simulink model "ctrl_student_HIL.previous"  (R2015a)
settings: Solver=ode4  StartTime=0.0  StopTime=inf  FixedStep=0.01  RelTol=1e-3
(part 3 of 3)

== matlab function ctrl_student_HIL.previous/Transfer function ==
  data: s input; eta input; nu input; mu input; rx input; ry input; kp1 input; kp2 input; kp3 input; s_dot output; tau output; eta_d output; case_number input
function [s_dot, tau, eta_d] = maneuver(s, eta, nu, mu, rx, ry, kp1, kp2, kp3, case_number)
%% Constants
P_d = [2 0; 10 4];
K_p = diag([kp1+0.2 kp2+0.2 kp3+0.1]);
K_2 = 10*eye(3); K_2(3, 3) = K_2(3, 3) / 2;
U_max = 0.6548;

%% Parameters
% Rigid body and added mass
m = 14.79; 
I_z = 1.76; 
x_g = 0.0375; 
% y_g = 0.0;

X_u_dot = -2; 
Y_v_dot = -10; 
Y_r_dot = -0; 
N_r_dot = -1; 

% Max Values in Surge X, Sway Y and Yaw N
X_max = 1.03; %[N]
Y_max = 2.50; %[N]
N_max = 0.98; %[Nm]


% Hydro surge, Hydro sway and Hydro Yaw Parameters
    % NB! We don't need most of them for now, that why they are commented
    % out, but don't remove them!!
X_u = -0.6555;  Y_v = -1.33;    N_v = 0.0; 
X_uu = 0.3545;  Y_vv = -2.776;  N_vv = -0.2088; 
X_uuu = -3.787; Y_vvv = -64.91; N_vvv = 0.0;
X_v = 0.0;      Y_r = -7.25;    N_r = -1.9; 
X_vv = -2.443;  Y_rr = -3.45;   N_rr = 0.75;
X_vvv = 0.0;    Y_rrr = 0.0;    N_rrr = 0.0;
                Y_rv = 0.805;   N_rv = 0.130;
                Y_vr = -0.845;  N_vr = 0.080;
      
% Matrices
u = nu(1); v = nu(2); r = nu(3); % I need a test values; 
    
a_11 = m-X_u_dot;   a_12 = 0;                   a_13 = 0; 
a_21 = 0;           a_22 = m-Y_v_dot ;          a_23 = m*x_g - Y_r_dot;
a_31 = 0;           a_32 = m*x_g - Y_r_dot;     a_33 = I_z - N_r_dot;

M = [a_11 a_12, a_13; a_12 a_22 a_23; a_31 a_32 a_33];

d_11_u =  -X_u - X_uu*abs(u) - X_uuu*u^2;
d_22_vr = -Y_v - Y_vv*abs(v) - Y_vvv*v^2   - Y_rv*abs(r);
d_23_vr = -Y_r - Y_vr*abs(v) - Y_rr*abs(r) - Y_rrr*r^2;
d_32_vr = -N_v - N_vv*abs(v) - N_vvv*v^2   - N_rv*abs(r);
d_33_vr = -N_r - N_vr*abs(v) - N_rr*abs(r) - N_rrr*r^2;

% The total damping matrix from the handbook page 53
D_tot = [d_11_u 0 0; 0 d_22_vr d_23_vr; 0 d_32_vr d_33_vr];

switch case_number
    case 1
        %% Straight line
        %% Speed mapping
        U_ref = U_max / 5;
        U_s = U_ref / sqrt(sum((P_d(:,2)-P_d(:,1)).^2));
        U_s_s = 0;

        %% Reference mapping
        p_d = max(min(s,1),0).*[P_d(2,1) - P_d(1,1); P_d(2,2) - P_d(1,2)] + [P_d(1,1); P_d(1,2)];
        psi_d = atan2(P_d(2,2) - P_d(1,2), P_d(2,1) - P_d(1,1));

        p_d_s = [P_d(2,1) - P_d(1,1); P_d(2,2) - P_d(1,2)];
        psi_d_s = 0;

        p_d_ss = [0; 0];
        psi_d_ss = 0;

        eta_d = [p_d; psi_d];
        eta_d_s = [p_d_s; psi_d_s];
        eta_d_ss = [p_d_ss; psi_d_ss];

        %% Update law
        diff = eta - eta_d; diff(3) = angdiff(eta_d(3), eta(3));
        if norm(eta_d_s) < 1e-5
            s_dot = U_s - mu * -diff' * ones(3,1) / norm(ones(3, 1));
        else
            s_dot = U_s - mu * -diff' * eta_d_s / norm(eta_d_s);
        end
        if s >= 1
            s_dot = 0;
            eta_d_s = eta_d_s*0;
        end
    case 2
        %% Forward and backward on a straight line
        %% Speed mapping
        U_ref = U_max / 5;
        U_s = U_ref / sqrt(sum((P_d(:,2)-P_d(:,1)).^2));
        U_s_s = 0;

        %% Reference mapping
        % These work, but go out of bounds below.
        multiplicant    = sin(s);
        derivicant      = cos(s);
        superderivicant = -sin(s);
        
        p_d = multiplicant*[P_d(2,1) - P_d(1,1); P_d(2,2) - P_d(1,2)]/2 + [P_d(2,1) - P_d(1,1); P_d(2,2) - P_d(1,2)]/2;
        psi_d = atan2(P_d(2,2) - P_d(1,2), P_d(2,1) - P_d(1,1));

        p_d_s = derivicant*[(P_d(2,1) - P_d(1,1)); (P_d(2,2) - P_d(1,2))]/2;
        psi_d_s = 0;

        p_d_ss = superderivicant*[(P_d(2,1) - P_d(1,1)); (P_d(2,2) - P_d(1,2))]/2;
        psi_d_ss = 0;

        eta_d = [p_d; psi_d];
        eta_d_s = [p_d_s; psi_d_s];
        eta_d_ss = [p_d_ss; psi_d_ss];

        %% Update law
        diff = eta - eta_d; diff(3) = angdiff(eta_d(3), eta(3));
        if norm(eta_d_s) < 1e-5
            s_dot = U_s - mu * -diff' * ones(3,1) / norm(ones(3, 1));
        else
            s_dot = U_s - mu * -diff' * eta_d_s / norm(eta_d_s);
        end
    case 3
        %% Forward and backward on a straight line with sinusoidal parametrization of U_ref
        %% Speed mapping
        U_ref = U_max / 5 * (1.01 + sin(2*pi*s - pi/2));
        U_s = U_ref / sqrt(sum((P_d(:,2)-P_d(:,1)).^2));
        U_s_s = 0;

        %% Reference mapping
        multiplicant    = sin(s);
        derivicant      = cos(s);
        superderivicant = -sin(s);
        
        p_d = multiplicant*[P_d(2,1) - P_d(1,1); P_d(2,2) - P_d(1,2)]/2 + [P_d(2,1) - P_d(1,1); P_d(2,2) - P_d(1,2)]/2;
        psi_d = atan2(P_d(2,2) - P_d(1,2), P_d(2,1) - P_d(1,1));

        p_d_s = derivicant*[(P_d(2,1) - P_d(1,1)); (P_d(2,2) - P_d(1,2))]/2;
        psi_d_s = 0;

        p_d_ss = superderivicant*[(P_d(2,1) - P_d(1,1)); (P_d(2,2) - P_d(1,2))]/2;
        psi_d_ss = 0;

        eta_d = [p_d; psi_d];
        eta_d_s = [p_d_s; psi_d_s];
        eta_d_ss = [p_d_ss; psi_d_ss];

        %% Update law
        diff = eta - eta_d; diff(3) = angdiff(eta_d(3), eta(3));
        if norm(eta_d_s) < 1e-5
            s_dot = U_s - mu * -diff' * ones(3,1) / norm(ones(3, 1));
        else
            s_dot = U_s - mu * -diff' * eta_d_s / norm(eta_d_s);
        end
    case 4
        %% Ellipse tracking
        C = [6; 0];
        
        %% Speed mapping
        % rx = 5;
        % ry = 3;
        U_ref = U_max / 10;
        U_s = U_ref / sqrt((rx*sin(s))^2 + (ry*cos(s))^2);
        U_s_s = -(rx^2*cos(s)*sin(s) - ry^2*cos(s)*sin(s))*U_ref/(ry^2*cos(s)^2 + rx^2*sin(s)^2)^(3/2);

        %% Reference mapping
        p_d = [rx*cos(s)+C(1); ry*sin(s)+C(2)];
        psi_d = atan2(ry*cos(s), -rx*sin(s));

        p_d_s = [-rx*sin(s); ry*cos(s)];
        psi_d_s = rx*ry/(ry^2*cos(s)^2+rx^2*sin(s)^2);

        p_d_ss = [-rx*cos(s); -ry*sin(s)];
        psi_d_ss = -2*(rx^2*cos(s)*sin(s) - ry^2*cos(s)*sin(s))*rx*ry/(ry^2*cos(s)^2 + rx^2*sin(s)^2)^2;

        eta_d = [p_d; psi_d];
        eta_d_s = [p_d_s; psi_d_s];
        eta_d_ss = [p_d_ss; psi_d_ss];

        %% Update law
        diff = eta - eta_d; diff(3) = angdiff(eta_d(3), eta(3));
        if norm(eta_d_s) < 1e-5
            s_dot = U_s - mu * -diff' * ones(3,1) / norm(ones(3, 1));
        else
            s_dot = U_s - mu * -diff' * eta_d_s / norm(eta_d_s);
        end
    otherwise
        %% Speed mapping
        U_ref = U_max / 5;
        U_s = U_ref;
        U_s_s = 0;

        %% Reference mapping
        p_d = [0; 0];
        psi_d = atan2(0 - eta(2), 0 - eta(1));

        p_d_s = [0; 0];
        psi_d_s = 0;

        p_d_ss = [0; 0];
        psi_d_ss = 0;

        eta_d = [p_d; psi_d];
        eta_d_s = [p_d_s; psi_d_s];
        eta_d_ss = [p_d_ss; psi_d_ss];

        %% Update law
        diff = eta - eta_d; diff(3) = angdiff(eta_d(3), eta(3));
        s_dot = 0;
end


%% Control law
% Define z_1 and z_1_dot
S = [0 -r 0; r 0 0; 0 0 0];
psi = eta(3);
R = [cos(psi) -sin(psi) 0;
     sin(psi) cos(psi)  0;
     0        0         1];
 
z_1_a = eta - eta_d;
z_1_psi = angdiff(eta_d(3), eta(3));
z_1_a(3) = z_1_psi;
z_1 = R'*z_1_a;
z_1_dot = S'*z_1 + nu - R'*eta_d_s*s_dot;

% alpha_1, alpha_1_dot, and z_2
alpha_1 = -K_p*z_1 + R'*eta_d_s*U_s;
z_2 = nu - alpha_1;
alpha_1_dot = -K_p*z_1_dot + S'*R'*eta_d_s*U_s + R'*eta_d_ss*s_dot*U_s + R'*eta_d_s*U_s_s*s_dot;

tau = D_tot*nu + M*alpha_1_dot - z_1 - K_2*z_2;
tau = prevent_boundary_break(eta, tau);
tau = min([X_max Y_max N_max]', tau);
tau = max(-[X_max Y_max N_max]', tau);

function diff = angdiff(alpha, beta)
diff = mod(beta - alpha + pi, 2*pi) - pi;

function tau_to_m = prevent_boundary_break(eta, tau)
limit = [-20 20; (-6.45/2) (6.45/2)]; % Axis in the middle of the pool (assumed)
percentage_x = 0.95;
percentage_y = 0.8;
a = percentage_x * limit(1, 2);
b = percentage_y * limit(2, 2);

tau_to_m = tau;
psi = eta(3);

R = [cos(psi) -sin(psi) 0;
     sin(psi) cos(psi)  0;
     0        0         1;];
norm4 = norm(eta(1:2)./[a b]', 4);
 
if norm4 > 1.0
    gradient = -[4/a*(eta(1)/a)^3 4/b*(eta(2)/b)^3]';
    tau_to_m(1:2) = gradient*10*(norm4 - 0.5);
    tau_to_m = R'*tau_to_m;
% This heuristic ensures that eta_d outside the basin
% will not immediately throttle the actuator towards eta_d once the
% vessel is back in the "safety zone" (norm4 < 1)
% We thus throttle the actuator forces down to avoid heavy
% oscillations.
elseif norm4 >= 0.90
    tau_to_m = tau*(1-norm4*0.75);
end

== matlab function ctrl_student_HIL.previous/Noise Generator/Noise generator/Sample & hold/MATLAB Function1 ==
  data: counter input; input input; hold input; output output
function output = fcn(counter,input,hold)
%#codegen

if counter == 0
    output = input;
else
    output = hold;
end

== matlab function ctrl_student_HIL.previous/Dead reckoning/MATLAB Function ==
  data: mem input; newmem output; eta_m input; dropout input; dead output
function [newmem, dead] = detect_dead_reckoning(mem, eta_m, dropout)
newmem = zeros(3, 1);
dead = zeros(3, 1);
for r = 1:3
    if eta_m(r) == mem(r) || dropout(r)
        dead(r) = 1;
        newmem(r) = mem(r);
    else
        newmem(r) = eta_m(r);
    end
end

== matlab function ctrl_student_HIL.previous/DP Observer /Observer  ==
  data: eta input; vec1 input; eta_hat_dot output; vec2 input; vec3 input; tau input; nu_hat_dot output; b_hat_dot output; x_bar output; eta_hat input; nu_hat input; b_hat input; y_bar output; psi_bar output; b input
function [eta_hat_dot, nu_hat_dot, b_hat_dot, x_bar, y_bar, psi_bar] = observer(eta, vec1, vec2, vec3, tau, eta_hat, nu_hat, b_hat, b)
% if(first == 1)
% eta_hat = zeros(3,1) ; 
% nu_hat = zeros(3,1); 
% b_hau = zeros(3,1)
% first_out = 0; 
% end
b = b + 2;
L1 = diag(vec1 + [4 4 3]'); 
L2 = diag(vec2 + [50 50 10]'); 
L3 = diag(vec3 + [20 20 10]'); 
M = [16.79 0 0; 0 24.79 0.5546; 0 0.5546 2.7600];



% The total damping matrix from the handbook page 53
D = [4.0880 0 0; 0 68.2110 0; 0 0.0788 1.070];


eta_bar = eta - eta_hat; 
x_bar = eta_bar(1); 
y_bar = eta_bar(2);
psi_bar = eta_bar(3); 
psi = eta(3); 
R = [cos(psi) sin(psi) 0; 
     -sin(psi) cos(psi) 0; 
     0 0 1]; 

nu_hat_dot = inv(M)*(-D*nu_hat + R'*b_hat + tau + R'*L2*eta_bar); 
eta_hat_dot = R*nu_hat + L1*eta_bar;

b_hat_dot = L3*eta_bar +b;

== matlab function ctrl_student_HIL.previous/SurgeObserver /Integration block  ==
  data: psi input; y output; k_0 input; X input; u_hat input; reset input
function y = fcn(psi, k_0, X,u_hat,reset)
a = sin(psi) + cos(psi); 
m_11 = 14.79; 

if reset
    u_hat=0;
end

if a < 0
k_psi = -k_0; 
else
k_psi = k_0; 
end

d_11 = 0.6555 - 0.3545*abs(u_hat) +3.787*(u_hat)^2; 

y = (-d_11*u_hat + X)/m_11 - k_psi*a*u_hat;

== matlab function ctrl_student_HIL.previous/SurgeObserver /the rest  ==
  data: x input; y input; psi input; k_0 input; y1 output
function y1 = fcn( x, y, psi, k_0)

a = sin(psi) + cos(psi); 

if a < 0
k_psi = -k_0; 
else
    k_psi = k_0; 
end

y1 = k_psi*(x + y)
